simulink model "mpc_pendcartNMPC"  (R2025a)
settings: Solver=ode15s  StartTime=0.0  StopTime=30  MaxStep=1e-3  RelTol=1e-3  EnableMultiTasking=on
values from neighbouring files (symbols this model uses):
  Ts = 0.1    [SwingupControlOfPendulumUsingNMPCExample.m]    (also in defineNonLiearMPCController.m)
libraries: mpclib x2, SignalEditorBlockLib x1, sharedTrackingLibrary x1
settings Model: Creator=The MathWorks, Inc.  LastModifiedBy=amyyang
settings SolverCC: AlgebraicLoopSolver=LineSearch
settings DataIOCC: LimitDataPoints=on  SaveFormat=Array  ReturnWorkspaceOutputs=off
settings OptimizationCC: ReuseModelBlockBuffer=off  LifeSpan=inf
settings DebuggingCC: AlgebraicLoopMsg=none  UnderspecifiedInitializationDetection=Classic  MergeDetectMultiDrivingBlocksExec=none  SolverPrmCheckMsg=warning  UnconnectedInputMsg=warning  UnconnectedOutputMsg=warning  UnconnectedLineMsg=warning  AllowSymbolicDim=off  StateNameClashWarn=warning  SFUnexpectedBacktrackingDiag=warning  SFNoUnconditionalDefaultTransitionDiag=warning  SFExecutionAtInitializationDiag=none  ArithmeticOperatorsInVariantConditions=warning
settings HardwareCC: ProdBitPerPointer=32.0  ProdBitPerSizeT=32.0  ProdBitPerPtrDiffT=32.0  ProdLargestAtomicFloat=None  ProdIntDivRoundTo=Undefined  ProdEndianess=Unspecified  ProdWordSize=32.0  ProdHWDeviceType=32-bit Generic
settings ModelReferenceCC: EnableRefExpFcnMdlSchedulingChecks=on  PropagateSignalLabelsOutOfModel=off
settings SFSimCC: SimUseLocalCustomCode=off  CustomCodeUndefinedFunction=UseInterfaceOnly
settings RTWCC: RTWUseLocalCustomCode=off  GPUComputeCapability=3.5  DLArmComputeVersion=19.05
settings CodeAppCC: StateflowObjectComments=on
settings GRTTargetCC: TargetLangStandard=C89/C90 (ANSI)
settings ConfigComp: CovMetricSettings=dw  CovSaveCumulativeToWorkspaceVar=on  CovSaveSingleToWorkspaceVar=on  CovExternalEMLEnable=off  CovSFcnEnable=off
settings SimscapeCC: SimscapeNormalizeSystem=off  SimscapeNominalValues="[{\"value\":\"10\",\"unit\":\"V\"},{\"value\":\"1\",\"unit\":\"A\"},{\"value\":\"10\",\"unit\":\"N*m\"},{\"value\":\"10\",\"unit\":\"bar\"},{\"value\":\"100\",\"unit\":\"kJ/kg\"},{\"value\":\"1\",\"unit\":\"kW\"},{\"value\":\"300\",\"unit\":\"K\"},{\"value\":\"100\",\"unit\":\"cm^3/s\"},{\"value\":\"1\",\"unit\":\"kN\"},{\"value\":\"1\",\"unit\":\"g/cm^3\"},{\"value\":\"1\",\"unit\":\"l\"},{\"value\":\"1\",\"unit\":\"cm^2\"},{\"value\":\"60\",\"unit\":\"Hz\"}]"
settings ConfigurationSet: Description=SimMechanics 2G
settings ExplorerConfigSet: InternalSimMechanicsExplorerSettings="<ExplorerConfiguration><canonicalview>default</canonicalview><AnimationSetting><BasePlaybackSpeed>1.0</BasePlaybackSpeed><PlaybackSpeedFactor>1.0</PlaybackSpeedFactor></AnimationSetting><TilePanel><TileInfo><Tiles Columns=\"1\" Count=\"1\" Rows=\"1\"><Column Left=\"2\" Weight=\"1\"/><Column Left=\"1552\"/><Row Top=\"2\" Weight=\"1\"/><Row Top=\"932\"/><Tile Height=\"1\" Width=\"1\" X=\"0\" Y=\"0\"/></Tiles></TileInfo><SceneInfo><SceneViewer><BGColor><R>0.60000002384185791</R><G>0.60000002384185791</G><B>0.60000002384185791</B></BGColor><Camera><Position><X>0.027865189060748197</X><Y>-2.5719092456962986</Y><Z>0.23157896538506753</Z></Position><Center><X>0.62659712312732463</X><Y>-0.46110119691712204</Y><Z>0.22087365386473376</Z></Center><Up><X>-0.0079438354874226333</X><Y>0.0073246425924307582</Y><Z>0.99994162084025784</Z></Up><Left>-0.24533778208815546</Left><Right>0.24533778208815546</Right><Bottom>-0.79734779727023208</Bottom><Top>0.79734779727023208</Top></Camera></SceneViewer></SceneInfo></TilePanel></ExplorerConfiguration>"

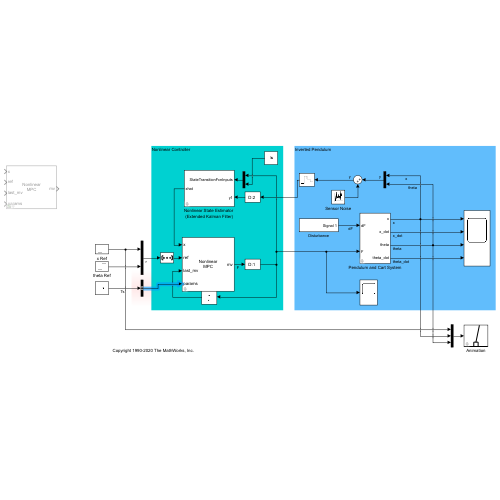
[thumbnail: Simulink's stored preview of the top-level diagram]
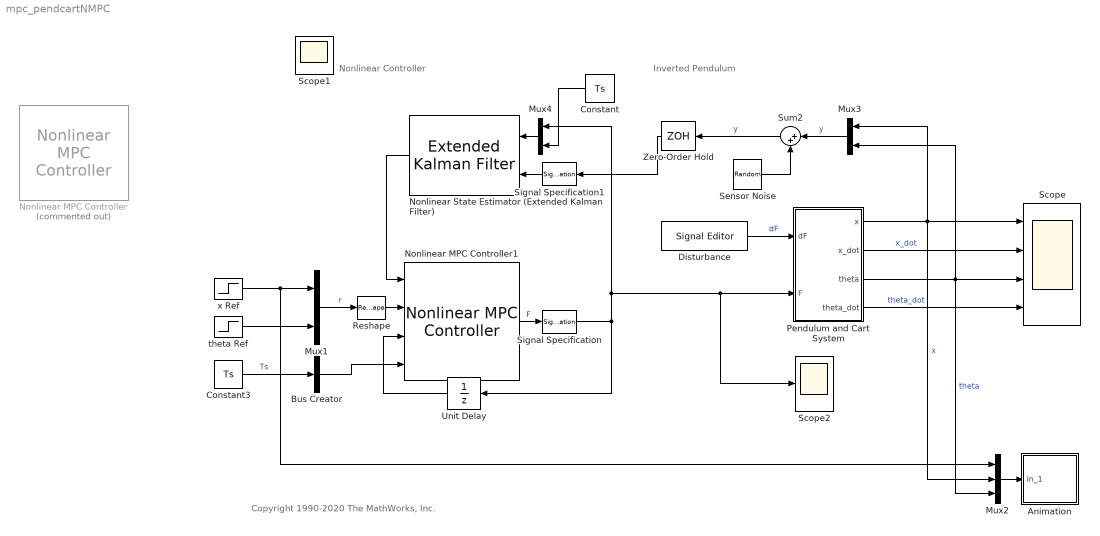
== system mpc_pendcartNMPC ==
  note: Nonlinear Controller
  note: Copyright 1990-2020 The MathWorks, Inc.
  note: Inverted Pendulum
  Animation : Subsystem  mask(Pendulum plot){RefBlock=x Ref}
      mask prompts: RefBlock "Cart Reference Signal Block Name:"
      mask help: Pendulum plot
      mask Help: Pendulum animation function using Handle graphics.
      mask Display: plot([-10 10],[0 0],[-2 -2 2 2],[0 1 1 0],[0 3],[1 5])
  Bus Creator : BusCreator  Inputs=1  OutDataTypeStr=Bus: myBusObject  NonVirtualBus=on
      settings: InheritFromInputs=off
  Constant : Constant  Value=Ts
  Constant3 : Constant  Value=Ts
  Disturbance : SignalEditorBlockLib/Signal Editor  FileName=pendulumDisturbance.mat  ActiveScenario=Group_1  ActiveSignal=Signal 1  IsBus=off  OutputBusObjectStr=Bus: BusObject  SampleTime=0  OutputAfterFinalValue=Extrapolation  Unit=inherit  PreserveSignalName=on  ApplySigPropsToAllScenarios=on  ApplySigPropsToAllSignals=off  SignalPropertySource=Dialog parameters
  Mux1 : Mux  Inputs=2
  Mux2 : Mux  Inputs=3
  Mux3 : Mux  Inputs=2
  Mux4 : Mux  Inputs=2
  Nonlinear MPC Controller : mpclib/Nonlinear MPC Controller  Commented=on  SCDEnableBlockLinearizationSpecification=on  nlmpcobj=nlobj  UseObjectTs=on  UseMEX=off  md_enabled=off  mvtarget_enabled=off  param_enabled=on  cost_enabled=off  mvseq_enabled=off  stateseq_enabled=off  ovseq_enabled=off  slack_enabled=off  status_enabled=off  ov_min=off  ov_max=off  mv_min=off  mv_max=off  mvrate_min=off  mvrate_max=off  state_min=off  state_max=off  ov_weight=off  mv_weight=off  mvrate_weight=off  ecr_weight=off  nlp_initialize=off
  Nonlinear MPC Controller1 : mpclib/Nonlinear MPC Controller  nlmpcobj=nlobj  UseObjectTs=on  UseMEX=off  md_enabled=off  mvtarget_enabled=off  param_enabled=on  cost_enabled=off  mvseq_enabled=off  stateseq_enabled=off  ovseq_enabled=off  slack_enabled=off  status_enabled=off  ov_min=off  ov_max=off  mv_min=off  mv_max=off  mvrate_min=off  mvrate_max=off  state_min=off  state_max=off  ov_weight=off  mv_weight=off  mvrate_weight=off  ecr_weight=off  nlp_initialize=off
  Nonlinear State Estimator (Extended Kalman Filter) : sharedTrackingLibrary/Extended Kalman Filter  StateTransitionFcn=pendulumStateFcn  HasStateTransitionJacobianFcn=off  HasAdditiveProcessNoise=Additive  ProcessNoise=1e-4*eye(4)  HasTimeVaryingProcessNoise=off  HasStateTransitionFcnExtraArgument=1  InitialState=[0;0;-pi;0]  InitialStateCovariance=1e-4*eye(4)  MeasurementFcn1=pendulumMeasurementFcn  HasMeasurementJacobianFcn1=off  HasMeasurementEnablePort1=off  HasAdditiveMeasurementNoise1=Additive  MeasurementNoise1=1e-4*eye(2)  HasTimeVaryingMeasurementNoise1=off  HasMeasurementFcnExtraArgument1=0  HasMeasurementWrapping1=off  MeasurementFcn2=myMeasurementFcn  HasMeasurementJacobianFcn2=off  HasMeasurementEnablePort2=off  HasAdditiveMeasurementNoise2=Additive  MeasurementNoise2=1  HasTimeVaryingMeasurementNoise2=off  HasMeasurementFcnExtraArgument2=0  HasMeasurementWrapping2=off  MeasurementFcn3=myMeasurementFcn  HasMeasurementJacobianFcn3=off  HasMeasurementEnablePort3=off  HasAdditiveMeasurementNoise3=Additive  MeasurementNoise3=1  HasTimeVaryingMeasurementNoise3=off  HasMeasurementFcnExtraArgument3=0  HasMeasurementWrapping3=off  MeasurementFcn4=myMeasurementFcn  HasMeasurementJacobianFcn4=off  HasMeasurementEnablePort4=off  HasAdditiveMeasurementNoise4=Additive  MeasurementNoise4=1  HasTimeVaryingMeasurementNoise4=off  HasMeasurementFcnExtraArgument4=0  HasMeasurementWrapping4=off  MeasurementFcn5=myMeasurementFcn  HasMeasurementJacobianFcn5=off  HasMeasurementEnablePort5=off  HasAdditiveMeasurementNoise5=Additive  MeasurementNoise5=1  HasTimeVaryingMeasurementNoise5=off  HasMeasurementFcnExtraArgument5=0  HasMeasurementWrapping5=off  EnableMultirate=off  StateTransitionFcnSampleTime=1  MeasurementFcn1SampleTime=1  MeasurementFcn2SampleTime=1  MeasurementFcn3SampleTime=1  MeasurementFcn4SampleTime=1  MeasurementFcn5SampleTime=1  UseCurrentEstimator=on  OutputStateCovariance=off  DataType=double  SampleTime=Ts  NumberOfMeasurements=1
  Pendulum and Cart System : Subsystem  mask{MCart=1, m=1, g=9.81, l=0.5, Kd=10, x0=0, theta0=-pi}
      mask prompts: MCart "Cart mass (Kg)"; m "Pendulum mass (Kg)"; g "Gravity (m/s^2)"; l "Distance from joint to pendulum center of mass (m)"; Kd "Viscous friction coefficient on cart (N*s/m)"; x0 "Initial cart position (m)"; theta0 "Initial pendulum angle (rad)"
      mask help:
      | Pendulum and Cart System
      |
      | The block represents a pendulum attached to an unactuated revolutionary joint on a cart, which moves along a one-dimensional track subject to viscous damping.
      |
      | The block inputs are the force F on the cart and the force dF on the pendulum. The block outputs are the four system states: linear position and velocity or the cart (rightward-positive), angular position and velocity of the pendulum (counterclockwise-positive, with the upright position being zero radians).
      |
      | Look under the mask to see the equations and their Simulink implementation. For a derivation of the system equations, click Help.
      mask Help: web('https://www.mathworks.com/help/symbolic/derive-and-simulate-cart-pole-system.html')
  Reshape : Reshape  OutputDimensionality=Row vector (2-D)
  Scope : Scope  NumInputPorts=4
      settings: ActiveDisplayYMinimum=-1.904  ActiveDisplayYMaximum=5.84249
  Scope2 : Scope
      settings: ActiveDisplayYMinimum=-122.4308  ActiveDisplayYMaximum=124.71453
  Sensor Noise : UniformRandomNumber  Minimum=-0.01  Maximum=0.01  SampleTime=Ts
  Signal Specification : SignalSpecification  Dimensions=1
  Signal Specification1 : SignalSpecification  Dimensions=2
  Sum2 : Sum  Inputs=|++
  Unit Delay : UnitDelay  SampleTime=-1  HasFrameUpgradeWarning=on
  Zero-Order Hold : ZeroOrderHold  SampleTime=Ts
  theta Ref : Step  Before=-pi  After=0  SampleTime=0
  x Ref : Step  Time=10  Before=0.67889  After=5  SampleTime=0
  Scope1 : Scope
      settings: ActiveDisplayYMinimum=-117.88073  ActiveDisplayYMaximum=60.92653  DataLoggingMaxPoints=7500  DataLoggingSaveFormat=Array
  wires:
  theta Ref/1 -> Mux1/2
  Pendulum and Cart System/4(theta_dot) -> Scope/4  "theta_dot"
  Pendulum and Cart System/2(x_dot) -> Scope/2  "x_dot"
  Disturbance/1 -> Pendulum and Cart System/1(dF)  "dF"
  Nonlinear MPC Controller1/1 -> Signal Specification/1  "F"
  Mux2/1 -> Animation/1(in_1)
  x Ref/1 -> Mux2/1, Mux1/1
  Unit Delay/1 -> Nonlinear MPC Controller1/3
  Mux3/1 -> Sum2/1  "y"
  Sensor Noise/1 -> Sum2/2
  Pendulum and Cart System/3(theta) -> Mux3/2, Mux2/3, Scope/3  "theta"
  Sum2/1 -> Zero-Order Hold/1  "y"
  Pendulum and Cart System/1(x) -> Mux3/1, Mux2/2, Scope/1  "x"
  Zero-Order Hold/1 -> Signal Specification1/1
  Mux4/1 -> Nonlinear State Estimator (Extended Kalman Filter)/1
  Constant/1 -> Mux4/2
  Nonlinear State Estimator (Extended Kalman Filter)/1 -> Nonlinear MPC Controller1/1
  Mux1/1 -> Reshape/1  "r"
  Reshape/1 -> Nonlinear MPC Controller1/2
  Constant3/1 -> Bus Creator/1  "Ts"
  Bus Creator/1 -> Nonlinear MPC Controller1/4
  Signal Specification/1 -> Unit Delay/1, Pendulum and Cart System/2(F), Scope2/1, Mux4/1
  Signal Specification1/1 -> Nonlinear State Estimator (Extended Kalman Filter)/2

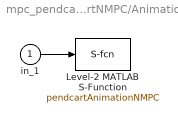
== system mpc_pendcartNMPC/Animation ==
  in_1 : Inport
  Level-2 MATLAB S-Function : M-S-Function  FunctionName=pendcartAnimationNMPC  Parameters=RefBlock
  wires:
  in_1/1 -> Level-2 MATLAB S-Function/1

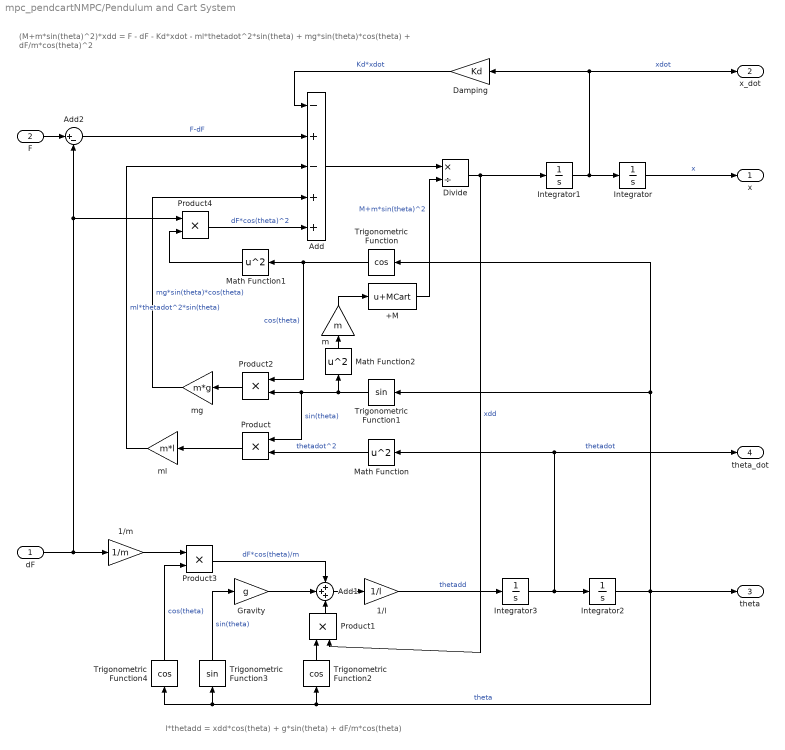
== system mpc_pendcartNMPC/Pendulum and Cart System ==
  note: l*thetadd = xdd*cos(theta) + g*sin(theta) + dF/m*cos(theta)
  note: (M+m*sin(theta)^2)*xdd = F - dF - Kd*xdot - ml*thetadot^2*sin(theta) + mg*sin(theta)*cos(theta) + dF/m*cos(theta)^2
  dF : Inport
  F : Inport  Port=2
  +M : Bias  Bias=MCart  SaturateOnIntegerOverflow=off
  1/l : Gain  Gain=1/l
  1/m : Gain  Gain=1/m
  Add : Sum  Inputs=-+-++
  Add1 : Sum  Inputs=+++
  Add2 : Sum  Inputs=|+-
  Damping : Gain  Gain=Kd
  Divide : Product  Inputs=*/
  Gravity : Gain  Gain=g
  Integrator : Integrator  InitialCondition=x0  ContinuousStateAttributes='x'
  Integrator1 : Integrator  ContinuousStateAttributes='xdot'
  Integrator2 : Integrator  InitialCondition=theta0  ContinuousStateAttributes='theta'
  Integrator3 : Integrator  ContinuousStateAttributes='thetadot'
  Math Function : Math  Operator=square  SignedPower=on
  Math Function1 : Math  Operator=square  SignedPower=on
  Math Function2 : Math  Operator=square  SignedPower=on
  Product{,1..4} (5 alike) : Product
  Trigonometric Function : Trigonometry  Operator=cos
  Trigonometric Function1 : Trigonometry
  Trigonometric Function2 : Trigonometry  Operator=cos
  Trigonometric Function3 : Trigonometry
  Trigonometric Function4 : Trigonometry  Operator=cos
  m : Gain  Gain=m
  mg : Gain  Gain=m*g
  ml : Gain  Gain=m*l
  x : Outport  VectorParamsAs1DForOutWhenUnconnected=off
  x_dot : Outport  Port=2  VectorParamsAs1DForOutWhenUnconnected=off
  theta : Outport  Port=3  VectorParamsAs1DForOutWhenUnconnected=off
  theta_dot : Outport  Port=4  VectorParamsAs1DForOutWhenUnconnected=off
  wires:
  Product/1 -> ml/1
  ml/1 -> Add/3  "ml*thetadot^2*sin(theta)"
  Add2/1 -> Add/2  "F-dF"
  Add1/1 -> 1/l/1
  Product2/1 -> mg/1
  Integrator1/1 -> Damping/1, x_dot/1, Integrator/1  "xdot"
  Integrator/1 -> x/1  "x"
  Trigonometric Function1/1 -> Math Function2/1, Product2/2, Product/1  "sin(theta)"
  Trigonometric Function2/1 -> Product1/1
  Divide/1 -> Integrator1/1, Product1/2  "xdd"
  Add/1 -> Divide/1
  Product3/1 -> Add1/1  "dF*cos(theta)/m"
  Integrator2/1 -> Trigonometric Function2/1, Trigonometric Function4/1, Trigonometric Function3/1, theta/1, Trigonometric Function1/1, Trigonometric Function/1  "theta"
  Integrator3/1 -> theta_dot/1, Math Function/1, Integrator2/1  "thetadot"
  Trigonometric Function/1 -> Product2/1, Math Function1/1  "cos(theta)"
  Gravity/1 -> Add1/2
  Trigonometric Function3/1 -> Gravity/1  "sin(theta)"
  F/1 -> Add2/1
  Damping/1 -> Add/1  "Kd*xdot"
  Trigonometric Function4/1 -> Product3/2  "cos(theta)"
  1/m/1 -> Product3/1
  dF/1 -> Product4/1, Add2/2, 1/m/1
  1/l/1 -> Integrator3/1  "thetadd"
  Math Function/1 -> Product/2  "thetadot^2"
  Product1/1 -> Add1/3
  mg/1 -> Add/4  "mg*sin(theta)*cos(theta)"
  Math Function1/1 -> Product4/2
  Product4/1 -> Add/5  "dF*cos(theta)^2"
  Math Function2/1 -> m/1
  +M/1 -> Divide/2  "M+m*sin(theta)^2"
  m/1 -> +M/1
